simulink model "randomAccessQueueTest_wQueue_wControllerClass"  (R2018b)
settings: Solver=VariableStepAuto  StartTime=0.0  StopTime=1000  RelTol=1e-3
undefined symbols (not defined in the file): m, n
settings Model: Creator=tas5  LastModifiedBy=tas5

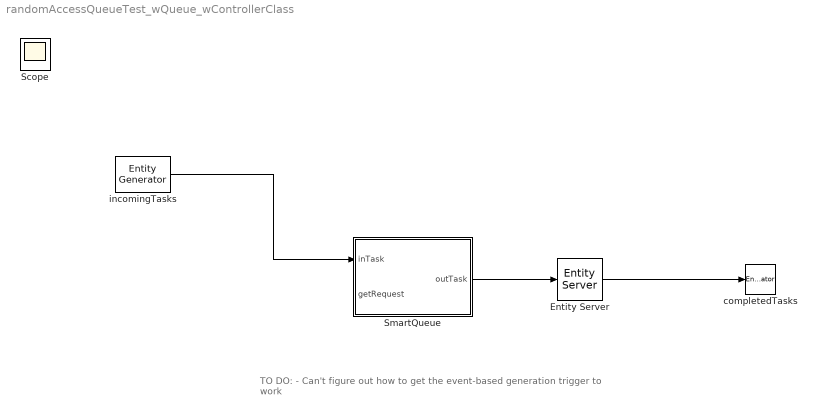
== system randomAccessQueueTest_wQueue_wControllerClass ==
  note: TO DO:
      | - Can't figure out how to get the event-based generation trigger to work
  Entity Server : EntityServer  InputPortMessageModes=m  OutputPortMessageModes=m  Capacity=1
  SmartQueue : Subsystem  InitFcn=|
      | coder.extrinsic('evalin')
      | 
      | evalin('base', 'availableTasks = []')
      | evalin('base', 'completedTasks = []')
      | 
      | evalin('base', 'QueueController = Controller;')
      | evalin('base', 'sq1 = RandomSequencing;')
      | evalin('base','QueueController.Sequencing = sq1;');
  completedTasks : EntityTerminator  InputPortMessageModes=m  EntryAction=|
      | coder.extrinsic('evalin');
      | coder.extrinsic('assignin');
      | coder.extrinsic('now');
      | 
      | %Read the queue list from workspace, then write new entity to it
      | %Return to workspace
      | completedTasks = evalin('base', 'completedTasks');
      | completedTasks = [completedTasks; [now, entity.ID, entity.Type, entity.Color]]
      | assignin('base', 'completedTasks', completedTasks)
  incomingTasks : EntityGenerator  OutputPortMessageModes=m  IntergenerationTimeAction=|  GenerateAction=|  AttributeName=ID|Type|Color|Priority  AttributeInitialValue=1|1|1|0  EntityType=Structured  EntityTypeName=Entity
      IntergenerationTimeAction=|
      | dt = rand(1,1);
      | persistent rngInit;
      | if isempty(rngInit)
      |     seed = 12345;
      |     rng(seed);
      |     rngInit = true;
      | end
      | 
      | % Pattern: Exponential distribution
      | mu = 1;
      | dt = -mu * log(1 - rand());
      GenerateAction=|
      | persistent idx
      | if isempty(idx)
      |     idx = 1;
      | end
      | 
      | %Colors = {'Red', 'Yellow', 'Blue'}
      | coder.extrinsic('randi')
      | 
      | entity.ID = idx;
      | entity.Type = randi(5,1);
      | entity.Color = randi(3,1);
      | 
      | idx = idx +1
  Scope : Scope
  wires:
  incomingTasks/1 -> SmartQueue/1(inTask)
  SmartQueue/1(outTask) -> Entity Server/1
  Entity Server/1 -> completedTasks/1

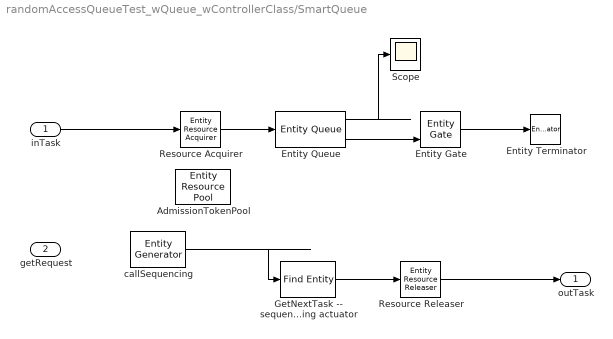
== system randomAccessQueueTest_wQueue_wControllerClass/SmartQueue ==
  inTask : Inport
  getRequest : Inport  Port=2
  AdmissionTokenPool : EntityResourcePool  ResourceName=AdmissionToken  ResourceAmount=100
  Entity Gate : EntityGate  InputPortMessageModes=m,m  OutputPortMessageModes=m
  Entity Queue : EntityQueue  InputPortMessageModes=m  OutputPortMessageModes=n,m  EntryAction=|  AverageWait=on
      | coder.extrinsic('evalin');
      | coder.extrinsic('assignin');
      | coder.extrinsic('now');
      | 
      | %Read the queue list from workspace, then write new entity to it
      | %Return to workspace
      | availableTasks = evalin('base', 'availableTasks');
      | availableTasks = [availableTasks; [0, now, entity.ID, entity.Type, entity.Color]]
      | assignin('base', 'availableTasks', availableTasks)
      settings: OutputPortMap=o2,o5
  Entity Terminator : EntityTerminator  InputPortMessageModes=m
  "GetNextTask -- sequencing actuator" : FindEntity  InputPortMessageModes=m  OutputPortMessageModes=m  ResourceName=AdmissionToken  EnableOutput=on  EntityFilter=on  MatchingCondition=|  NumberEntitiesFound=on
      | %coder.extrinsic('evalin')
      | %index = evalin('base', 'Sequencing(availableTasks);')
      | %match = isequal(index, entity.ID);
      | 
      | match = isequal(trigger.selectedID, entity.ID);
      settings: OutputPortMap=o6
  Resource Acquirer : EntityResourceAcquirer  InputPortMessageModes=m  OutputPortMessageModes=m  NumberWaitingEntities=100  ResourceName=AdmissionToken
      settings: OutputPortMap=o3
  Resource Releaser : EntityResourceReleaser  InputPortMessageModes=m  OutputPortMessageModes=m  ResourceToRelease=Selected  ResourceName=AdmissionToken
  Scope : Scope
  callSequencing : EntityGenerator  OutputPortMessageModes=m  Period=2  GenerateEntityAtSimulationStart=off  GenerateAction=|  AttributeName=selectedID  EntityType=Structured  EntityTypeName=trigger  EntityPriority=100
      | coder.extrinsic('evalin')
      | %coder.extrinsic('assignin')
      | %coder.extrinsic('sortrows')
      | %coder.extrinsic('min')
      | %coder.extrinsic('Sequencing')
      | 
      | entity.selectedID = evalin('base', 'QueueController.Sequencing.Sequencing(availableTasks);')
      | 
      | 
      | %queuedEntity = evalin('base', 'queuedEntity');
      | %call sequencing
      | %[B,I] = sortrows(queuedEntity, [4,5,2]);
      | %queuedEntity(:,1) = I;
      | %[Y, J] = min(I);
      | %assignin('base','queuedEntity', B);
      | %evalin('base', 'queuedEntity(1,:) = []');
      | %entity.selectedID = queuedEntity(J,3);
  outTask : Outport
  wires:
  callSequencing/1 -> "GetNextTask -- sequencing actuator"/1
  inTask/1 -> Resource Acquirer/1
  "GetNextTask -- sequencing actuator"/1 -> Resource Releaser/1
  Resource Releaser/1 -> outTask/1
  Entity Queue/2 -> Entity Gate/2
  Entity Gate/1 -> Entity Terminator/1
  Resource Acquirer/1 -> Entity Queue/1
  Entity Queue/1 -> Scope/1
